simulink model "fft_wideband_real"  (R2012b)
settings: Solver=ode45  StartTime=0.0  StopTime=19999  RelTol=1e-3
undefined symbols (not defined in the file): fft_wideband_real_shift_schedule_user_data_out
libraries: xbsIndex_r4 x8703, xbsReplacements_r4 x36, xps_library x24, dspsigops x16, simulink_xsg_bridge x1
(part 7 of 51)

== system fft_wideband_real/fft_wideband_real/phase_mult/cmult_1 ==
  a : Inport
  b : Inport  Port=2
  AddSub : xbsIndex_r4/AddSub  mode=Subtraction  use_carryin=off  use_carryout=off  en=off  latency=2  precision=Full  arith_type=Unsigned  n_bits=16  bin_pt=14  quantization=Truncate  overflow=Wrap  dbl_ovrd=off  use_behavioral_HDL=on  hw_selection=Fabric  pipelined=off  block_type=addsub
  AddSub1 : xbsIndex_r4/AddSub  mode=Addition  use_carryin=off  use_carryout=off  en=off  latency=2  precision=Full  arith_type=Unsigned  n_bits=16  bin_pt=14  quantization=Truncate  overflow=Wrap  dbl_ovrd=off  use_behavioral_HDL=on  hw_selection=Fabric  pipelined=off  block_type=addsub
  a_input_c_to_ri : Subsystem
      settings: AttributesFormatString=18_17 r/i
  b_input_c_to_ri : Subsystem
      settings: AttributesFormatString=18_17 r/i
  c_output_ri_to_c : Subsystem
  convert0 : xbsIndex_r4/Convert  gui_display_data_type=Fixed-point  arith_type="Signed  (2's comp)"  n_bits=18  bin_pt=17  float_type=Single  exp_bits=8  fraction_bits=24  quantization="Round  (unbiased: +/- Inf)"  overflow=Saturate  en=off  latency=1  dbl_ovrd=off  pipeline=on  block_type=convert
  convert1 : xbsIndex_r4/Convert  gui_display_data_type=Fixed-point  arith_type="Signed  (2's comp)"  n_bits=18  bin_pt=17  float_type=Single  exp_bits=8  fraction_bits=24  quantization="Round  (unbiased: +/- Inf)"  overflow=Saturate  en=off  latency=1  dbl_ovrd=off  pipeline=on  block_type=convert
  mults : Subsystem
  c : Outport
  wires:
  a_input_c_to_ri/1(re) -> mults/7(a4), mults/1(a1)  "a_re"
  b_input_c_to_ri/1(re) -> mults/6(b3), mults/2(b1)  "b_re"
  a_input_c_to_ri/2(im) -> mults/5(a3), mults/3(a2)  "a_im"
  b_input_c_to_ri/2(im) -> mults/8(b4), mults/4(b2)  "b_im"
  convert1/1 -> c_output_ri_to_c/2(im)  "c_im"
  AddSub1/1 -> convert1/1
  convert0/1 -> c_output_ri_to_c/1(re)  "c_re"
  AddSub/1 -> convert0/1
  mults/4(c4) -> AddSub1/2
  mults/3(c3) -> AddSub1/1
  mults/2(c2) -> AddSub/2
  mults/1(c1) -> AddSub/1
  c_output_ri_to_c/1(c) -> c/1
  b/1 -> b_input_c_to_ri/1(c)
  a/1 -> a_input_c_to_ri/1(c)

== system fft_wideband_real/fft_wideband_real/phase_mult/cmult_10 ==
  a : Inport
  b : Inport  Port=2
  AddSub : xbsIndex_r4/AddSub  mode=Subtraction  use_carryin=off  use_carryout=off  en=off  latency=2  precision=Full  arith_type=Unsigned  n_bits=16  bin_pt=14  quantization=Truncate  overflow=Wrap  dbl_ovrd=off  use_behavioral_HDL=on  hw_selection=Fabric  pipelined=off  block_type=addsub
  AddSub1 : xbsIndex_r4/AddSub  mode=Addition  use_carryin=off  use_carryout=off  en=off  latency=2  precision=Full  arith_type=Unsigned  n_bits=16  bin_pt=14  quantization=Truncate  overflow=Wrap  dbl_ovrd=off  use_behavioral_HDL=on  hw_selection=Fabric  pipelined=off  block_type=addsub
  a_input_c_to_ri : Subsystem
      settings: AttributesFormatString=18_17 r/i
  b_input_c_to_ri : Subsystem
      settings: AttributesFormatString=18_17 r/i
  c_output_ri_to_c : Subsystem
  convert0 : xbsIndex_r4/Convert  gui_display_data_type=Fixed-point  arith_type="Signed  (2's comp)"  n_bits=18  bin_pt=17  float_type=Single  exp_bits=8  fraction_bits=24  quantization="Round  (unbiased: +/- Inf)"  overflow=Saturate  en=off  latency=1  dbl_ovrd=off  pipeline=on  block_type=convert
  convert1 : xbsIndex_r4/Convert  gui_display_data_type=Fixed-point  arith_type="Signed  (2's comp)"  n_bits=18  bin_pt=17  float_type=Single  exp_bits=8  fraction_bits=24  quantization="Round  (unbiased: +/- Inf)"  overflow=Saturate  en=off  latency=1  dbl_ovrd=off  pipeline=on  block_type=convert
  mults : Subsystem
  c : Outport
  wires:
  a_input_c_to_ri/1(re) -> mults/7(a4), mults/1(a1)  "a_re"
  b_input_c_to_ri/1(re) -> mults/6(b3), mults/2(b1)  "b_re"
  a_input_c_to_ri/2(im) -> mults/5(a3), mults/3(a2)  "a_im"
  b_input_c_to_ri/2(im) -> mults/8(b4), mults/4(b2)  "b_im"
  convert1/1 -> c_output_ri_to_c/2(im)  "c_im"
  AddSub1/1 -> convert1/1
  convert0/1 -> c_output_ri_to_c/1(re)  "c_re"
  AddSub/1 -> convert0/1
  mults/4(c4) -> AddSub1/2
  mults/3(c3) -> AddSub1/1
  mults/2(c2) -> AddSub/2
  mults/1(c1) -> AddSub/1
  c_output_ri_to_c/1(c) -> c/1
  b/1 -> b_input_c_to_ri/1(c)
  a/1 -> a_input_c_to_ri/1(c)

== system fft_wideband_real/fft_wideband_real/phase_mult/cmult_11 ==
  a : Inport
  b : Inport  Port=2
  AddSub : xbsIndex_r4/AddSub  mode=Subtraction  use_carryin=off  use_carryout=off  en=off  latency=2  precision=Full  arith_type=Unsigned  n_bits=16  bin_pt=14  quantization=Truncate  overflow=Wrap  dbl_ovrd=off  use_behavioral_HDL=on  hw_selection=Fabric  pipelined=off  block_type=addsub
  AddSub1 : xbsIndex_r4/AddSub  mode=Addition  use_carryin=off  use_carryout=off  en=off  latency=2  precision=Full  arith_type=Unsigned  n_bits=16  bin_pt=14  quantization=Truncate  overflow=Wrap  dbl_ovrd=off  use_behavioral_HDL=on  hw_selection=Fabric  pipelined=off  block_type=addsub
  a_input_c_to_ri : Subsystem
      settings: AttributesFormatString=18_17 r/i
  b_input_c_to_ri : Subsystem
      settings: AttributesFormatString=18_17 r/i
  c_output_ri_to_c : Subsystem
  convert0 : xbsIndex_r4/Convert  gui_display_data_type=Fixed-point  arith_type="Signed  (2's comp)"  n_bits=18  bin_pt=17  float_type=Single  exp_bits=8  fraction_bits=24  quantization="Round  (unbiased: +/- Inf)"  overflow=Saturate  en=off  latency=1  dbl_ovrd=off  pipeline=on  block_type=convert
  convert1 : xbsIndex_r4/Convert  gui_display_data_type=Fixed-point  arith_type="Signed  (2's comp)"  n_bits=18  bin_pt=17  float_type=Single  exp_bits=8  fraction_bits=24  quantization="Round  (unbiased: +/- Inf)"  overflow=Saturate  en=off  latency=1  dbl_ovrd=off  pipeline=on  block_type=convert
  mults : Subsystem
  c : Outport
  wires:
  a_input_c_to_ri/1(re) -> mults/7(a4), mults/1(a1)  "a_re"
  b_input_c_to_ri/1(re) -> mults/6(b3), mults/2(b1)  "b_re"
  a_input_c_to_ri/2(im) -> mults/5(a3), mults/3(a2)  "a_im"
  b_input_c_to_ri/2(im) -> mults/8(b4), mults/4(b2)  "b_im"
  convert1/1 -> c_output_ri_to_c/2(im)  "c_im"
  AddSub1/1 -> convert1/1
  convert0/1 -> c_output_ri_to_c/1(re)  "c_re"
  AddSub/1 -> convert0/1
  mults/4(c4) -> AddSub1/2
  mults/3(c3) -> AddSub1/1
  mults/2(c2) -> AddSub/2
  mults/1(c1) -> AddSub/1
  c_output_ri_to_c/1(c) -> c/1
  b/1 -> b_input_c_to_ri/1(c)
  a/1 -> a_input_c_to_ri/1(c)

== system fft_wideband_real/fft_wideband_real/phase_mult/cmult_12 ==
  a : Inport
  b : Inport  Port=2
  AddSub : xbsIndex_r4/AddSub  mode=Subtraction  use_carryin=off  use_carryout=off  en=off  latency=2  precision=Full  arith_type=Unsigned  n_bits=16  bin_pt=14  quantization=Truncate  overflow=Wrap  dbl_ovrd=off  use_behavioral_HDL=on  hw_selection=Fabric  pipelined=off  block_type=addsub
  AddSub1 : xbsIndex_r4/AddSub  mode=Addition  use_carryin=off  use_carryout=off  en=off  latency=2  precision=Full  arith_type=Unsigned  n_bits=16  bin_pt=14  quantization=Truncate  overflow=Wrap  dbl_ovrd=off  use_behavioral_HDL=on  hw_selection=Fabric  pipelined=off  block_type=addsub
  a_input_c_to_ri : Subsystem
      settings: AttributesFormatString=18_17 r/i
  b_input_c_to_ri : Subsystem
      settings: AttributesFormatString=18_17 r/i
  c_output_ri_to_c : Subsystem
  convert0 : xbsIndex_r4/Convert  gui_display_data_type=Fixed-point  arith_type="Signed  (2's comp)"  n_bits=18  bin_pt=17  float_type=Single  exp_bits=8  fraction_bits=24  quantization="Round  (unbiased: +/- Inf)"  overflow=Saturate  en=off  latency=1  dbl_ovrd=off  pipeline=on  block_type=convert
  convert1 : xbsIndex_r4/Convert  gui_display_data_type=Fixed-point  arith_type="Signed  (2's comp)"  n_bits=18  bin_pt=17  float_type=Single  exp_bits=8  fraction_bits=24  quantization="Round  (unbiased: +/- Inf)"  overflow=Saturate  en=off  latency=1  dbl_ovrd=off  pipeline=on  block_type=convert
  mults : Subsystem
  c : Outport
  wires:
  a_input_c_to_ri/1(re) -> mults/7(a4), mults/1(a1)  "a_re"
  b_input_c_to_ri/1(re) -> mults/6(b3), mults/2(b1)  "b_re"
  a_input_c_to_ri/2(im) -> mults/5(a3), mults/3(a2)  "a_im"
  b_input_c_to_ri/2(im) -> mults/8(b4), mults/4(b2)  "b_im"
  convert1/1 -> c_output_ri_to_c/2(im)  "c_im"
  AddSub1/1 -> convert1/1
  convert0/1 -> c_output_ri_to_c/1(re)  "c_re"
  AddSub/1 -> convert0/1
  mults/4(c4) -> AddSub1/2
  mults/3(c3) -> AddSub1/1
  mults/2(c2) -> AddSub/2
  mults/1(c1) -> AddSub/1
  c_output_ri_to_c/1(c) -> c/1
  b/1 -> b_input_c_to_ri/1(c)
  a/1 -> a_input_c_to_ri/1(c)

== system fft_wideband_real/fft_wideband_real/phase_mult/cmult_13 ==
  a : Inport
  b : Inport  Port=2
  AddSub : xbsIndex_r4/AddSub  mode=Subtraction  use_carryin=off  use_carryout=off  en=off  latency=2  precision=Full  arith_type=Unsigned  n_bits=16  bin_pt=14  quantization=Truncate  overflow=Wrap  dbl_ovrd=off  use_behavioral_HDL=on  hw_selection=Fabric  pipelined=off  block_type=addsub
  AddSub1 : xbsIndex_r4/AddSub  mode=Addition  use_carryin=off  use_carryout=off  en=off  latency=2  precision=Full  arith_type=Unsigned  n_bits=16  bin_pt=14  quantization=Truncate  overflow=Wrap  dbl_ovrd=off  use_behavioral_HDL=on  hw_selection=Fabric  pipelined=off  block_type=addsub
  a_input_c_to_ri : Subsystem
      settings: AttributesFormatString=18_17 r/i
  b_input_c_to_ri : Subsystem
      settings: AttributesFormatString=18_17 r/i
  c_output_ri_to_c : Subsystem
  convert0 : xbsIndex_r4/Convert  gui_display_data_type=Fixed-point  arith_type="Signed  (2's comp)"  n_bits=18  bin_pt=17  float_type=Single  exp_bits=8  fraction_bits=24  quantization="Round  (unbiased: +/- Inf)"  overflow=Saturate  en=off  latency=1  dbl_ovrd=off  pipeline=on  block_type=convert
  convert1 : xbsIndex_r4/Convert  gui_display_data_type=Fixed-point  arith_type="Signed  (2's comp)"  n_bits=18  bin_pt=17  float_type=Single  exp_bits=8  fraction_bits=24  quantization="Round  (unbiased: +/- Inf)"  overflow=Saturate  en=off  latency=1  dbl_ovrd=off  pipeline=on  block_type=convert
  mults : Subsystem
  c : Outport
  wires:
  a_input_c_to_ri/1(re) -> mults/7(a4), mults/1(a1)  "a_re"
  b_input_c_to_ri/1(re) -> mults/6(b3), mults/2(b1)  "b_re"
  a_input_c_to_ri/2(im) -> mults/5(a3), mults/3(a2)  "a_im"
  b_input_c_to_ri/2(im) -> mults/8(b4), mults/4(b2)  "b_im"
  convert1/1 -> c_output_ri_to_c/2(im)  "c_im"
  AddSub1/1 -> convert1/1
  convert0/1 -> c_output_ri_to_c/1(re)  "c_re"
  AddSub/1 -> convert0/1
  mults/4(c4) -> AddSub1/2
  mults/3(c3) -> AddSub1/1
  mults/2(c2) -> AddSub/2
  mults/1(c1) -> AddSub/1
  c_output_ri_to_c/1(c) -> c/1
  b/1 -> b_input_c_to_ri/1(c)
  a/1 -> a_input_c_to_ri/1(c)

== system fft_wideband_real/fft_wideband_real/phase_mult/cmult_14 ==
  a : Inport
  b : Inport  Port=2
  AddSub : xbsIndex_r4/AddSub  mode=Subtraction  use_carryin=off  use_carryout=off  en=off  latency=2  precision=Full  arith_type=Unsigned  n_bits=16  bin_pt=14  quantization=Truncate  overflow=Wrap  dbl_ovrd=off  use_behavioral_HDL=on  hw_selection=Fabric  pipelined=off  block_type=addsub
  AddSub1 : xbsIndex_r4/AddSub  mode=Addition  use_carryin=off  use_carryout=off  en=off  latency=2  precision=Full  arith_type=Unsigned  n_bits=16  bin_pt=14  quantization=Truncate  overflow=Wrap  dbl_ovrd=off  use_behavioral_HDL=on  hw_selection=Fabric  pipelined=off  block_type=addsub
  a_input_c_to_ri : Subsystem
      settings: AttributesFormatString=18_17 r/i
  b_input_c_to_ri : Subsystem
      settings: AttributesFormatString=18_17 r/i
  c_output_ri_to_c : Subsystem
  convert0 : xbsIndex_r4/Convert  gui_display_data_type=Fixed-point  arith_type="Signed  (2's comp)"  n_bits=18  bin_pt=17  float_type=Single  exp_bits=8  fraction_bits=24  quantization="Round  (unbiased: +/- Inf)"  overflow=Saturate  en=off  latency=1  dbl_ovrd=off  pipeline=on  block_type=convert
  convert1 : xbsIndex_r4/Convert  gui_display_data_type=Fixed-point  arith_type="Signed  (2's comp)"  n_bits=18  bin_pt=17  float_type=Single  exp_bits=8  fraction_bits=24  quantization="Round  (unbiased: +/- Inf)"  overflow=Saturate  en=off  latency=1  dbl_ovrd=off  pipeline=on  block_type=convert
  mults : Subsystem
  c : Outport
  wires:
  a_input_c_to_ri/1(re) -> mults/7(a4), mults/1(a1)  "a_re"
  b_input_c_to_ri/1(re) -> mults/6(b3), mults/2(b1)  "b_re"
  a_input_c_to_ri/2(im) -> mults/5(a3), mults/3(a2)  "a_im"
  b_input_c_to_ri/2(im) -> mults/8(b4), mults/4(b2)  "b_im"
  convert1/1 -> c_output_ri_to_c/2(im)  "c_im"
  AddSub1/1 -> convert1/1
  convert0/1 -> c_output_ri_to_c/1(re)  "c_re"
  AddSub/1 -> convert0/1
  mults/4(c4) -> AddSub1/2
  mults/3(c3) -> AddSub1/1
  mults/2(c2) -> AddSub/2
  mults/1(c1) -> AddSub/1
  c_output_ri_to_c/1(c) -> c/1
  b/1 -> b_input_c_to_ri/1(c)
  a/1 -> a_input_c_to_ri/1(c)

== system fft_wideband_real/fft_wideband_real/phase_mult/cmult_15 ==
  a : Inport
  b : Inport  Port=2
  AddSub : xbsIndex_r4/AddSub  mode=Subtraction  use_carryin=off  use_carryout=off  en=off  latency=2  precision=Full  arith_type=Unsigned  n_bits=16  bin_pt=14  quantization=Truncate  overflow=Wrap  dbl_ovrd=off  use_behavioral_HDL=on  hw_selection=Fabric  pipelined=off  block_type=addsub
  AddSub1 : xbsIndex_r4/AddSub  mode=Addition  use_carryin=off  use_carryout=off  en=off  latency=2  precision=Full  arith_type=Unsigned  n_bits=16  bin_pt=14  quantization=Truncate  overflow=Wrap  dbl_ovrd=off  use_behavioral_HDL=on  hw_selection=Fabric  pipelined=off  block_type=addsub
  a_input_c_to_ri : Subsystem
      settings: AttributesFormatString=18_17 r/i
  b_input_c_to_ri : Subsystem
      settings: AttributesFormatString=18_17 r/i
  c_output_ri_to_c : Subsystem
  convert0 : xbsIndex_r4/Convert  gui_display_data_type=Fixed-point  arith_type="Signed  (2's comp)"  n_bits=18  bin_pt=17  float_type=Single  exp_bits=8  fraction_bits=24  quantization="Round  (unbiased: +/- Inf)"  overflow=Saturate  en=off  latency=1  dbl_ovrd=off  pipeline=on  block_type=convert
  convert1 : xbsIndex_r4/Convert  gui_display_data_type=Fixed-point  arith_type="Signed  (2's comp)"  n_bits=18  bin_pt=17  float_type=Single  exp_bits=8  fraction_bits=24  quantization="Round  (unbiased: +/- Inf)"  overflow=Saturate  en=off  latency=1  dbl_ovrd=off  pipeline=on  block_type=convert
  mults : Subsystem
  c : Outport
  wires:
  a_input_c_to_ri/1(re) -> mults/7(a4), mults/1(a1)  "a_re"
  b_input_c_to_ri/1(re) -> mults/6(b3), mults/2(b1)  "b_re"
  a_input_c_to_ri/2(im) -> mults/5(a3), mults/3(a2)  "a_im"
  b_input_c_to_ri/2(im) -> mults/8(b4), mults/4(b2)  "b_im"
  convert1/1 -> c_output_ri_to_c/2(im)  "c_im"
  AddSub1/1 -> convert1/1
  convert0/1 -> c_output_ri_to_c/1(re)  "c_re"
  AddSub/1 -> convert0/1
  mults/4(c4) -> AddSub1/2
  mults/3(c3) -> AddSub1/1
  mults/2(c2) -> AddSub/2
  mults/1(c1) -> AddSub/1
  c_output_ri_to_c/1(c) -> c/1
  b/1 -> b_input_c_to_ri/1(c)
  a/1 -> a_input_c_to_ri/1(c)

== system fft_wideband_real/fft_wideband_real/phase_mult/cmult_16 ==
  a : Inport
  b : Inport  Port=2
  AddSub : xbsIndex_r4/AddSub  mode=Subtraction  use_carryin=off  use_carryout=off  en=off  latency=2  precision=Full  arith_type=Unsigned  n_bits=16  bin_pt=14  quantization=Truncate  overflow=Wrap  dbl_ovrd=off  use_behavioral_HDL=on  hw_selection=Fabric  pipelined=off  block_type=addsub
  AddSub1 : xbsIndex_r4/AddSub  mode=Addition  use_carryin=off  use_carryout=off  en=off  latency=2  precision=Full  arith_type=Unsigned  n_bits=16  bin_pt=14  quantization=Truncate  overflow=Wrap  dbl_ovrd=off  use_behavioral_HDL=on  hw_selection=Fabric  pipelined=off  block_type=addsub
  a_input_c_to_ri : Subsystem
      settings: AttributesFormatString=18_17 r/i
  b_input_c_to_ri : Subsystem
      settings: AttributesFormatString=18_17 r/i
  c_output_ri_to_c : Subsystem
  convert0 : xbsIndex_r4/Convert  gui_display_data_type=Fixed-point  arith_type="Signed  (2's comp)"  n_bits=18  bin_pt=17  float_type=Single  exp_bits=8  fraction_bits=24  quantization="Round  (unbiased: +/- Inf)"  overflow=Saturate  en=off  latency=1  dbl_ovrd=off  pipeline=on  block_type=convert
  convert1 : xbsIndex_r4/Convert  gui_display_data_type=Fixed-point  arith_type="Signed  (2's comp)"  n_bits=18  bin_pt=17  float_type=Single  exp_bits=8  fraction_bits=24  quantization="Round  (unbiased: +/- Inf)"  overflow=Saturate  en=off  latency=1  dbl_ovrd=off  pipeline=on  block_type=convert
  mults : Subsystem
  c : Outport
  wires:
  a_input_c_to_ri/1(re) -> mults/7(a4), mults/1(a1)  "a_re"
  b_input_c_to_ri/1(re) -> mults/6(b3), mults/2(b1)  "b_re"
  a_input_c_to_ri/2(im) -> mults/5(a3), mults/3(a2)  "a_im"
  b_input_c_to_ri/2(im) -> mults/8(b4), mults/4(b2)  "b_im"
  convert1/1 -> c_output_ri_to_c/2(im)  "c_im"
  AddSub1/1 -> convert1/1
  convert0/1 -> c_output_ri_to_c/1(re)  "c_re"
  AddSub/1 -> convert0/1
  mults/4(c4) -> AddSub1/2
  mults/3(c3) -> AddSub1/1
  mults/2(c2) -> AddSub/2
  mults/1(c1) -> AddSub/1
  c_output_ri_to_c/1(c) -> c/1
  b/1 -> b_input_c_to_ri/1(c)
  a/1 -> a_input_c_to_ri/1(c)

== system fft_wideband_real/fft_wideband_real/phase_mult/cmult_2 ==
  a : Inport
  b : Inport  Port=2
  AddSub : xbsIndex_r4/AddSub  mode=Subtraction  use_carryin=off  use_carryout=off  en=off  latency=2  precision=Full  arith_type=Unsigned  n_bits=16  bin_pt=14  quantization=Truncate  overflow=Wrap  dbl_ovrd=off  use_behavioral_HDL=on  hw_selection=Fabric  pipelined=off  block_type=addsub
  AddSub1 : xbsIndex_r4/AddSub  mode=Addition  use_carryin=off  use_carryout=off  en=off  latency=2  precision=Full  arith_type=Unsigned  n_bits=16  bin_pt=14  quantization=Truncate  overflow=Wrap  dbl_ovrd=off  use_behavioral_HDL=on  hw_selection=Fabric  pipelined=off  block_type=addsub
  a_input_c_to_ri : Subsystem
      settings: AttributesFormatString=18_17 r/i
  b_input_c_to_ri : Subsystem
      settings: AttributesFormatString=18_17 r/i
  c_output_ri_to_c : Subsystem
  convert0 : xbsIndex_r4/Convert  gui_display_data_type=Fixed-point  arith_type="Signed  (2's comp)"  n_bits=18  bin_pt=17  float_type=Single  exp_bits=8  fraction_bits=24  quantization="Round  (unbiased: +/- Inf)"  overflow=Saturate  en=off  latency=1  dbl_ovrd=off  pipeline=on  block_type=convert
  convert1 : xbsIndex_r4/Convert  gui_display_data_type=Fixed-point  arith_type="Signed  (2's comp)"  n_bits=18  bin_pt=17  float_type=Single  exp_bits=8  fraction_bits=24  quantization="Round  (unbiased: +/- Inf)"  overflow=Saturate  en=off  latency=1  dbl_ovrd=off  pipeline=on  block_type=convert
  mults : Subsystem
  c : Outport
  wires:
  a_input_c_to_ri/1(re) -> mults/7(a4), mults/1(a1)  "a_re"
  b_input_c_to_ri/1(re) -> mults/6(b3), mults/2(b1)  "b_re"
  a_input_c_to_ri/2(im) -> mults/5(a3), mults/3(a2)  "a_im"
  b_input_c_to_ri/2(im) -> mults/8(b4), mults/4(b2)  "b_im"
  convert1/1 -> c_output_ri_to_c/2(im)  "c_im"
  AddSub1/1 -> convert1/1
  convert0/1 -> c_output_ri_to_c/1(re)  "c_re"
  AddSub/1 -> convert0/1
  mults/4(c4) -> AddSub1/2
  mults/3(c3) -> AddSub1/1
  mults/2(c2) -> AddSub/2
  mults/1(c1) -> AddSub/1
  c_output_ri_to_c/1(c) -> c/1
  b/1 -> b_input_c_to_ri/1(c)
  a/1 -> a_input_c_to_ri/1(c)

== system fft_wideband_real/fft_wideband_real/phase_mult/cmult_3 ==
  a : Inport
  b : Inport  Port=2
  AddSub : xbsIndex_r4/AddSub  mode=Subtraction  use_carryin=off  use_carryout=off  en=off  latency=2  precision=Full  arith_type=Unsigned  n_bits=16  bin_pt=14  quantization=Truncate  overflow=Wrap  dbl_ovrd=off  use_behavioral_HDL=on  hw_selection=Fabric  pipelined=off  block_type=addsub
  AddSub1 : xbsIndex_r4/AddSub  mode=Addition  use_carryin=off  use_carryout=off  en=off  latency=2  precision=Full  arith_type=Unsigned  n_bits=16  bin_pt=14  quantization=Truncate  overflow=Wrap  dbl_ovrd=off  use_behavioral_HDL=on  hw_selection=Fabric  pipelined=off  block_type=addsub
  a_input_c_to_ri : Subsystem
      settings: AttributesFormatString=18_17 r/i
  b_input_c_to_ri : Subsystem
      settings: AttributesFormatString=18_17 r/i
  c_output_ri_to_c : Subsystem
  convert0 : xbsIndex_r4/Convert  gui_display_data_type=Fixed-point  arith_type="Signed  (2's comp)"  n_bits=18  bin_pt=17  float_type=Single  exp_bits=8  fraction_bits=24  quantization="Round  (unbiased: +/- Inf)"  overflow=Saturate  en=off  latency=1  dbl_ovrd=off  pipeline=on  block_type=convert
  convert1 : xbsIndex_r4/Convert  gui_display_data_type=Fixed-point  arith_type="Signed  (2's comp)"  n_bits=18  bin_pt=17  float_type=Single  exp_bits=8  fraction_bits=24  quantization="Round  (unbiased: +/- Inf)"  overflow=Saturate  en=off  latency=1  dbl_ovrd=off  pipeline=on  block_type=convert
  mults : Subsystem
  c : Outport
  wires:
  a_input_c_to_ri/1(re) -> mults/7(a4), mults/1(a1)  "a_re"
  b_input_c_to_ri/1(re) -> mults/6(b3), mults/2(b1)  "b_re"
  a_input_c_to_ri/2(im) -> mults/5(a3), mults/3(a2)  "a_im"
  b_input_c_to_ri/2(im) -> mults/8(b4), mults/4(b2)  "b_im"
  convert1/1 -> c_output_ri_to_c/2(im)  "c_im"
  AddSub1/1 -> convert1/1
  convert0/1 -> c_output_ri_to_c/1(re)  "c_re"
  AddSub/1 -> convert0/1
  mults/4(c4) -> AddSub1/2
  mults/3(c3) -> AddSub1/1
  mults/2(c2) -> AddSub/2
  mults/1(c1) -> AddSub/1
  c_output_ri_to_c/1(c) -> c/1
  b/1 -> b_input_c_to_ri/1(c)
  a/1 -> a_input_c_to_ri/1(c)

== system fft_wideband_real/fft_wideband_real/phase_mult/cmult_4 ==
  a : Inport
  b : Inport  Port=2
  AddSub : xbsIndex_r4/AddSub  mode=Subtraction  use_carryin=off  use_carryout=off  en=off  latency=2  precision=Full  arith_type=Unsigned  n_bits=16  bin_pt=14  quantization=Truncate  overflow=Wrap  dbl_ovrd=off  use_behavioral_HDL=on  hw_selection=Fabric  pipelined=off  block_type=addsub
  AddSub1 : xbsIndex_r4/AddSub  mode=Addition  use_carryin=off  use_carryout=off  en=off  latency=2  precision=Full  arith_type=Unsigned  n_bits=16  bin_pt=14  quantization=Truncate  overflow=Wrap  dbl_ovrd=off  use_behavioral_HDL=on  hw_selection=Fabric  pipelined=off  block_type=addsub
  a_input_c_to_ri : Subsystem
      settings: AttributesFormatString=18_17 r/i
  b_input_c_to_ri : Subsystem
      settings: AttributesFormatString=18_17 r/i
  c_output_ri_to_c : Subsystem
  convert0 : xbsIndex_r4/Convert  gui_display_data_type=Fixed-point  arith_type="Signed  (2's comp)"  n_bits=18  bin_pt=17  float_type=Single  exp_bits=8  fraction_bits=24  quantization="Round  (unbiased: +/- Inf)"  overflow=Saturate  en=off  latency=1  dbl_ovrd=off  pipeline=on  block_type=convert
  convert1 : xbsIndex_r4/Convert  gui_display_data_type=Fixed-point  arith_type="Signed  (2's comp)"  n_bits=18  bin_pt=17  float_type=Single  exp_bits=8  fraction_bits=24  quantization="Round  (unbiased: +/- Inf)"  overflow=Saturate  en=off  latency=1  dbl_ovrd=off  pipeline=on  block_type=convert
  mults : Subsystem
  c : Outport
  wires:
  a_input_c_to_ri/1(re) -> mults/7(a4), mults/1(a1)  "a_re"
  b_input_c_to_ri/1(re) -> mults/6(b3), mults/2(b1)  "b_re"
  a_input_c_to_ri/2(im) -> mults/5(a3), mults/3(a2)  "a_im"
  b_input_c_to_ri/2(im) -> mults/8(b4), mults/4(b2)  "b_im"
  convert1/1 -> c_output_ri_to_c/2(im)  "c_im"
  AddSub1/1 -> convert1/1
  convert0/1 -> c_output_ri_to_c/1(re)  "c_re"
  AddSub/1 -> convert0/1
  mults/4(c4) -> AddSub1/2
  mults/3(c3) -> AddSub1/1
  mults/2(c2) -> AddSub/2
  mults/1(c1) -> AddSub/1
  c_output_ri_to_c/1(c) -> c/1
  b/1 -> b_input_c_to_ri/1(c)
  a/1 -> a_input_c_to_ri/1(c)

== system fft_wideband_real/fft_wideband_real/phase_mult/cmult_5 ==
  a : Inport
  b : Inport  Port=2
  AddSub : xbsIndex_r4/AddSub  mode=Subtraction  use_carryin=off  use_carryout=off  en=off  latency=2  precision=Full  arith_type=Unsigned  n_bits=16  bin_pt=14  quantization=Truncate  overflow=Wrap  dbl_ovrd=off  use_behavioral_HDL=on  hw_selection=Fabric  pipelined=off  block_type=addsub
  AddSub1 : xbsIndex_r4/AddSub  mode=Addition  use_carryin=off  use_carryout=off  en=off  latency=2  precision=Full  arith_type=Unsigned  n_bits=16  bin_pt=14  quantization=Truncate  overflow=Wrap  dbl_ovrd=off  use_behavioral_HDL=on  hw_selection=Fabric  pipelined=off  block_type=addsub
  a_input_c_to_ri : Subsystem
      settings: AttributesFormatString=18_17 r/i
  b_input_c_to_ri : Subsystem
      settings: AttributesFormatString=18_17 r/i
  c_output_ri_to_c : Subsystem
  convert0 : xbsIndex_r4/Convert  gui_display_data_type=Fixed-point  arith_type="Signed  (2's comp)"  n_bits=18  bin_pt=17  float_type=Single  exp_bits=8  fraction_bits=24  quantization="Round  (unbiased: +/- Inf)"  overflow=Saturate  en=off  latency=1  dbl_ovrd=off  pipeline=on  block_type=convert
  convert1 : xbsIndex_r4/Convert  gui_display_data_type=Fixed-point  arith_type="Signed  (2's comp)"  n_bits=18  bin_pt=17  float_type=Single  exp_bits=8  fraction_bits=24  quantization="Round  (unbiased: +/- Inf)"  overflow=Saturate  en=off  latency=1  dbl_ovrd=off  pipeline=on  block_type=convert
  mults : Subsystem
  c : Outport
  wires:
  a_input_c_to_ri/1(re) -> mults/7(a4), mults/1(a1)  "a_re"
  b_input_c_to_ri/1(re) -> mults/6(b3), mults/2(b1)  "b_re"
  a_input_c_to_ri/2(im) -> mults/5(a3), mults/3(a2)  "a_im"
  b_input_c_to_ri/2(im) -> mults/8(b4), mults/4(b2)  "b_im"
  convert1/1 -> c_output_ri_to_c/2(im)  "c_im"
  AddSub1/1 -> convert1/1
  convert0/1 -> c_output_ri_to_c/1(re)  "c_re"
  AddSub/1 -> convert0/1
  mults/4(c4) -> AddSub1/2
  mults/3(c3) -> AddSub1/1
  mults/2(c2) -> AddSub/2
  mults/1(c1) -> AddSub/1
  c_output_ri_to_c/1(c) -> c/1
  b/1 -> b_input_c_to_ri/1(c)
  a/1 -> a_input_c_to_ri/1(c)

== system fft_wideband_real/fft_wideband_real/phase_mult/cmult_6 ==
  a : Inport
  b : Inport  Port=2
  AddSub : xbsIndex_r4/AddSub  mode=Subtraction  use_carryin=off  use_carryout=off  en=off  latency=2  precision=Full  arith_type=Unsigned  n_bits=16  bin_pt=14  quantization=Truncate  overflow=Wrap  dbl_ovrd=off  use_behavioral_HDL=on  hw_selection=Fabric  pipelined=off  block_type=addsub
  AddSub1 : xbsIndex_r4/AddSub  mode=Addition  use_carryin=off  use_carryout=off  en=off  latency=2  precision=Full  arith_type=Unsigned  n_bits=16  bin_pt=14  quantization=Truncate  overflow=Wrap  dbl_ovrd=off  use_behavioral_HDL=on  hw_selection=Fabric  pipelined=off  block_type=addsub
  a_input_c_to_ri : Subsystem
      settings: AttributesFormatString=18_17 r/i
  b_input_c_to_ri : Subsystem
      settings: AttributesFormatString=18_17 r/i
  c_output_ri_to_c : Subsystem
  convert0 : xbsIndex_r4/Convert  gui_display_data_type=Fixed-point  arith_type="Signed  (2's comp)"  n_bits=18  bin_pt=17  float_type=Single  exp_bits=8  fraction_bits=24  quantization="Round  (unbiased: +/- Inf)"  overflow=Saturate  en=off  latency=1  dbl_ovrd=off  pipeline=on  block_type=convert
  convert1 : xbsIndex_r4/Convert  gui_display_data_type=Fixed-point  arith_type="Signed  (2's comp)"  n_bits=18  bin_pt=17  float_type=Single  exp_bits=8  fraction_bits=24  quantization="Round  (unbiased: +/- Inf)"  overflow=Saturate  en=off  latency=1  dbl_ovrd=off  pipeline=on  block_type=convert
  mults : Subsystem
  c : Outport
  wires:
  a_input_c_to_ri/1(re) -> mults/7(a4), mults/1(a1)  "a_re"
  b_input_c_to_ri/1(re) -> mults/6(b3), mults/2(b1)  "b_re"
  a_input_c_to_ri/2(im) -> mults/5(a3), mults/3(a2)  "a_im"
  b_input_c_to_ri/2(im) -> mults/8(b4), mults/4(b2)  "b_im"
  convert1/1 -> c_output_ri_to_c/2(im)  "c_im"
  AddSub1/1 -> convert1/1
  convert0/1 -> c_output_ri_to_c/1(re)  "c_re"
  AddSub/1 -> convert0/1
  mults/4(c4) -> AddSub1/2
  mults/3(c3) -> AddSub1/1
  mults/2(c2) -> AddSub/2
  mults/1(c1) -> AddSub/1
  c_output_ri_to_c/1(c) -> c/1
  b/1 -> b_input_c_to_ri/1(c)
  a/1 -> a_input_c_to_ri/1(c)

== system fft_wideband_real/fft_wideband_real/phase_mult/cmult_7 ==
  a : Inport
  b : Inport  Port=2
  AddSub : xbsIndex_r4/AddSub  mode=Subtraction  use_carryin=off  use_carryout=off  en=off  latency=2  precision=Full  arith_type=Unsigned  n_bits=16  bin_pt=14  quantization=Truncate  overflow=Wrap  dbl_ovrd=off  use_behavioral_HDL=on  hw_selection=Fabric  pipelined=off  block_type=addsub
  AddSub1 : xbsIndex_r4/AddSub  mode=Addition  use_carryin=off  use_carryout=off  en=off  latency=2  precision=Full  arith_type=Unsigned  n_bits=16  bin_pt=14  quantization=Truncate  overflow=Wrap  dbl_ovrd=off  use_behavioral_HDL=on  hw_selection=Fabric  pipelined=off  block_type=addsub
  a_input_c_to_ri : Subsystem
      settings: AttributesFormatString=18_17 r/i
  b_input_c_to_ri : Subsystem
      settings: AttributesFormatString=18_17 r/i
  c_output_ri_to_c : Subsystem
  convert0 : xbsIndex_r4/Convert  gui_display_data_type=Fixed-point  arith_type="Signed  (2's comp)"  n_bits=18  bin_pt=17  float_type=Single  exp_bits=8  fraction_bits=24  quantization="Round  (unbiased: +/- Inf)"  overflow=Saturate  en=off  latency=1  dbl_ovrd=off  pipeline=on  block_type=convert
  convert1 : xbsIndex_r4/Convert  gui_display_data_type=Fixed-point  arith_type="Signed  (2's comp)"  n_bits=18  bin_pt=17  float_type=Single  exp_bits=8  fraction_bits=24  quantization="Round  (unbiased: +/- Inf)"  overflow=Saturate  en=off  latency=1  dbl_ovrd=off  pipeline=on  block_type=convert
  mults : Subsystem
  c : Outport
  wires:
  a_input_c_to_ri/1(re) -> mults/7(a4), mults/1(a1)  "a_re"
  b_input_c_to_ri/1(re) -> mults/6(b3), mults/2(b1)  "b_re"
  a_input_c_to_ri/2(im) -> mults/5(a3), mults/3(a2)  "a_im"
  b_input_c_to_ri/2(im) -> mults/8(b4), mults/4(b2)  "b_im"
  convert1/1 -> c_output_ri_to_c/2(im)  "c_im"
  AddSub1/1 -> convert1/1
  convert0/1 -> c_output_ri_to_c/1(re)  "c_re"
  AddSub/1 -> convert0/1
  mults/4(c4) -> AddSub1/2
  mults/3(c3) -> AddSub1/1
  mults/2(c2) -> AddSub/2
  mults/1(c1) -> AddSub/1
  c_output_ri_to_c/1(c) -> c/1
  b/1 -> b_input_c_to_ri/1(c)
  a/1 -> a_input_c_to_ri/1(c)

== system fft_wideband_real/fft_wideband_real/phase_mult/cmult_8 ==
  a : Inport
  b : Inport  Port=2
  AddSub : xbsIndex_r4/AddSub  mode=Subtraction  use_carryin=off  use_carryout=off  en=off  latency=2  precision=Full  arith_type=Unsigned  n_bits=16  bin_pt=14  quantization=Truncate  overflow=Wrap  dbl_ovrd=off  use_behavioral_HDL=on  hw_selection=Fabric  pipelined=off  block_type=addsub
  AddSub1 : xbsIndex_r4/AddSub  mode=Addition  use_carryin=off  use_carryout=off  en=off  latency=2  precision=Full  arith_type=Unsigned  n_bits=16  bin_pt=14  quantization=Truncate  overflow=Wrap  dbl_ovrd=off  use_behavioral_HDL=on  hw_selection=Fabric  pipelined=off  block_type=addsub
  a_input_c_to_ri : Subsystem
      settings: AttributesFormatString=18_17 r/i
  b_input_c_to_ri : Subsystem
      settings: AttributesFormatString=18_17 r/i
  c_output_ri_to_c : Subsystem
  convert0 : xbsIndex_r4/Convert  gui_display_data_type=Fixed-point  arith_type="Signed  (2's comp)"  n_bits=18  bin_pt=17  float_type=Single  exp_bits=8  fraction_bits=24  quantization="Round  (unbiased: +/- Inf)"  overflow=Saturate  en=off  latency=1  dbl_ovrd=off  pipeline=on  block_type=convert
  convert1 : xbsIndex_r4/Convert  gui_display_data_type=Fixed-point  arith_type="Signed  (2's comp)"  n_bits=18  bin_pt=17  float_type=Single  exp_bits=8  fraction_bits=24  quantization="Round  (unbiased: +/- Inf)"  overflow=Saturate  en=off  latency=1  dbl_ovrd=off  pipeline=on  block_type=convert
  mults : Subsystem
  c : Outport
  wires:
  a_input_c_to_ri/1(re) -> mults/7(a4), mults/1(a1)  "a_re"
  b_input_c_to_ri/1(re) -> mults/6(b3), mults/2(b1)  "b_re"
  a_input_c_to_ri/2(im) -> mults/5(a3), mults/3(a2)  "a_im"
  b_input_c_to_ri/2(im) -> mults/8(b4), mults/4(b2)  "b_im"
  convert1/1 -> c_output_ri_to_c/2(im)  "c_im"
  AddSub1/1 -> convert1/1
  convert0/1 -> c_output_ri_to_c/1(re)  "c_re"
  AddSub/1 -> convert0/1
  mults/4(c4) -> AddSub1/2
  mults/3(c3) -> AddSub1/1
  mults/2(c2) -> AddSub/2
  mults/1(c1) -> AddSub/1
  c_output_ri_to_c/1(c) -> c/1
  b/1 -> b_input_c_to_ri/1(c)
  a/1 -> a_input_c_to_ri/1(c)

== system fft_wideband_real/fft_wideband_real/phase_mult/cmult_9 ==
  a : Inport
  b : Inport  Port=2
  AddSub : xbsIndex_r4/AddSub  mode=Subtraction  use_carryin=off  use_carryout=off  en=off  latency=2  precision=Full  arith_type=Unsigned  n_bits=16  bin_pt=14  quantization=Truncate  overflow=Wrap  dbl_ovrd=off  use_behavioral_HDL=on  hw_selection=Fabric  pipelined=off  block_type=addsub
  AddSub1 : xbsIndex_r4/AddSub  mode=Addition  use_carryin=off  use_carryout=off  en=off  latency=2  precision=Full  arith_type=Unsigned  n_bits=16  bin_pt=14  quantization=Truncate  overflow=Wrap  dbl_ovrd=off  use_behavioral_HDL=on  hw_selection=Fabric  pipelined=off  block_type=addsub
  a_input_c_to_ri : Subsystem
      settings: AttributesFormatString=18_17 r/i
  b_input_c_to_ri : Subsystem
      settings: AttributesFormatString=18_17 r/i
  c_output_ri_to_c : Subsystem
  convert0 : xbsIndex_r4/Convert  gui_display_data_type=Fixed-point  arith_type="Signed  (2's comp)"  n_bits=18  bin_pt=17  float_type=Single  exp_bits=8  fraction_bits=24  quantization="Round  (unbiased: +/- Inf)"  overflow=Saturate  en=off  latency=1  dbl_ovrd=off  pipeline=on  block_type=convert
  convert1 : xbsIndex_r4/Convert  gui_display_data_type=Fixed-point  arith_type="Signed  (2's comp)"  n_bits=18  bin_pt=17  float_type=Single  exp_bits=8  fraction_bits=24  quantization="Round  (unbiased: +/- Inf)"  overflow=Saturate  en=off  latency=1  dbl_ovrd=off  pipeline=on  block_type=convert
  mults : Subsystem
  c : Outport
  wires:
  a_input_c_to_ri/1(re) -> mults/7(a4), mults/1(a1)  "a_re"
  b_input_c_to_ri/1(re) -> mults/6(b3), mults/2(b1)  "b_re"
  a_input_c_to_ri/2(im) -> mults/5(a3), mults/3(a2)  "a_im"
  b_input_c_to_ri/2(im) -> mults/8(b4), mults/4(b2)  "b_im"
  convert1/1 -> c_output_ri_to_c/2(im)  "c_im"
  AddSub1/1 -> convert1/1
  convert0/1 -> c_output_ri_to_c/1(re)  "c_re"
  AddSub/1 -> convert0/1
  mults/4(c4) -> AddSub1/2
  mults/3(c3) -> AddSub1/1
  mults/2(c2) -> AddSub/2
  mults/1(c1) -> AddSub/1
  c_output_ri_to_c/1(c) -> c/1
  b/1 -> b_input_c_to_ri/1(c)
  a/1 -> a_input_c_to_ri/1(c)

== system fft_wideband_real/fft_wideband_real/phase_mult/phase10_coeffs ==
  rst : Inport
  Counter : xbsIndex_r4/Counter  cnt_type=Free Running  cnt_to=Inf  operation=Up  start_count=0  cnt_by_val=1  arith_type=Unsigned  n_bits=6  bin_pt=0  load_pin=off  rst=on  en=off  explicit_period=on  period=1  dbl_ovrd=off  use_behavioral_HDL=off  implementation=Fabric  block_type=counter
  Slice : xbsIndex_r4/Slice  nbits=6  boolean_output=off  mode=Upper Bit Location + Width  bit1=0  base1=MSB of Input  bit0=0  base0=LSB of Input  dbl_ovrd=off  block_type=slice
  bram_din_const : xbsIndex_r4/Constant  const=0  gui_display_data_type=Fixed-point  arith_type=Signed (2's comp)  n_bits=18  bin_pt=17  preci_type=Single  exp_width=8  frac_width=24  explicit_period=off  period=1  equ=P=C  opselect=C  inp2=PCIN>>17  opr=+  inp1=P  carry=CIN  dbl_ovrd=off  block_type=constant
  bram_we_const : xbsIndex_r4/Constant  const=0  gui_display_data_type=Fixed-point  arith_type=Boolean  n_bits=16  bin_pt=14  preci_type=Single  exp_width=8  frac_width=24  explicit_period=off  period=1  equ=P=C  opselect=C  inp2=PCIN>>17  opr=+  inp1=P  carry=CIN  dbl_ovrd=off  block_type=constant
  cnt_sign_exta : xbsIndex_r4/Convert  gui_display_data_type=Fixed-point  arith_type=Unsigned  n_bits=10  bin_pt=0  float_type=Single  exp_bits=8  fraction_bits=24  quantization=Truncate  overflow=Wrap  en=off  latency=0  dbl_ovrd=off  pipeline=off  block_type=convert
  cnt_sign_extb : xbsIndex_r4/Convert  gui_display_data_type=Fixed-point  arith_type=Unsigned  n_bits=9  bin_pt=0  float_type=Single  exp_bits=8  fraction_bits=24  quantization=Truncate  overflow=Wrap  en=off  latency=0  dbl_ovrd=off  pipeline=off  block_type=convert
  coeff_mem : xbsIndex_r4/Dual Port RAM  depth=1024  initVector=[1 0.99847412109375 0.993904113769531 0.986305236816406 0.975700378417969 0.962120056152344 0.945610046386719 0.92620849609375 0.90399169921875 0.879013061523438 0.851356506347656 0.82110595703125 0.788345336914062 0.753189086914062 0.715728759765625 0.676094055175781 0.634391784667969 0.59075927734375 0.545326232910156 0.49822998046875 0.449607849121094 0.399627685546875 0.348419189453125 0.296150207519531 0.24298095703125 0.189071655273438 0.13458251953125 0.079681396484375 0.0245437622070312 -0.0306777954101562 -0.0858001708984375 -0.140655517578125 -0.195091247558594 -0.248924255371094 -0.302009582519531 -0.354164123535156 -0.405242919921875 -0.455085754394531 -0.5035400390625 -0.550460815429688 -0.595695495605469 -0.639122009277344 -0.68060302734375 -0.720001220703125 -0.757209777832031 -0.792106628417969 -0.824592590332031 -0.854560852050781 -0.881919860839844 -0.906593322753906 -0.928504943847656 -0.947586059570312 -0.963775634765625 -0.977027893066406 -0.9873046875 -0.99456787109375 -0.998794555664062 -0.999984741210938 -0.998115539550781 -0.993209838867188 -0.985275268554688 -0.974342346191406 -0.960433959960938 -0.943595886230469 0 0 0 0 0 0 0 0 0 0 0 0 0 0 0 0 0 0 0 0 0 0 0 0 0 0 0 0 0 0 0 0 0 0 0 0 0 0 0 0 0 0 0 0 0 0 0 0 0 0 0 0 0 0 0 0 0 0 0 0 0 0 0 0 0 0 0 0 0 0 0 0 0 0 0 0 0 0 0 0 0 0 0 0 0 0 0 0 0 0 0 0 0 0 0 0 0 0 0 0 0 0 0 0 0 0 0 0 0 0 0 0 0 0 0 0 0 0 0 0 0 0 0 0 0 0 0 0 0 0 0 0 0 0 0 0 0 0 0 0 0 0 0 0 0 0 0 0 0 0 0 0 0 0 0 0 0 0 0 0 0 0 0 0 0 0 0 0 0 0 0 0 0 0 0 0 0 0 0 0 0 0 0 0 0 0 0 0 0 0 0 0 0 0 0 0 0 0 0 0 0 0 0 0 0 0 0 0 0 0 0 0 0 0 0 0 0 0 0 0 0 0 0 0 0 0 0 0 0 0 0 0 0 0 0 0 0 0 0 0 0 0 0 0 0 0 0 0 0 0 0 0 0 0 0 0 0 0 0 0 0 0 0 0 0 0 0 0 0 0 0 0 0 0 0 0 0 0 0 0 0 0 0 0 0 0 0 0 0 0 0 0 0 0 0 0 0 0 0 0 0 0 0 0 0 0 0 0 0 0 0 0 0 0 0 0 0 0 0 0 0 0 0 0 0 0 0 0 0 0 0 0 0 0 0 0 0 0 0 0 0 0 0 0 0 0 0 0 0 0 0 0 0 0 0 0 0 0 0 0 0 0 0 0 0 0 0 0 0 0 0 0 0 0 0 0 0 0 0 0 0 0 0 0 0 0 0 0 0 0 0 0 0 0 0 0 0 0 0 0 0 0 0 0 0 0 0 0 0 0 0 0 0 0 0 0 0 0 0 0 0 0 0 0 0 0 0 0 0 0 0 0 0 0 0 0 0 0 0 0 0 0 0 0 0 0 0 0 0 -0.0551986694335938 -0.110221862792969 -0.164909362792969 -0.219100952148438 -0.272621154785156 -0.325309753417969 -0.377006530761719 -0.427558898925781 -0.476799011230469 -0.524589538574219 -0.570777893066406 -0.615234375 -0.657806396484375 -0.698379516601562 -0.73681640625 -0.77301025390625 -0.806846618652344 -0.838226318359375 -0.867042541503906 -0.893226623535156 -0.916679382324219 -0.937339782714844 -0.95513916015625 -0.97003173828125 -0.981964111328125 -0.99090576171875 -0.996818542480469 -0.999702453613281 -0.999526977539062 -0.996315002441406 -0.990058898925781 -0.980781555175781 -0.968521118164062 -0.95330810546875 -0.9351806640625 -0.914207458496094 -0.890449523925781 -0.863975524902344 -0.834861755371094 -0.803207397460938 -0.76910400390625 -0.732650756835938 -0.6939697265625 -0.653175354003906 -0.610382080078125 -0.56573486328125 -0.519355773925781 -0.471397399902344 -0.4219970703125 -0.371315002441406 -0.319503784179688 -0.266716003417969 -0.213111877441406 -0.158859252929688 -0.104118347167969 -0.0490646362304688 0.006134033203125 0.0613174438476562 0.116317749023438 0.17095947265625 0.225082397460938 0.278518676757812 0.331108093261719 0 0 0 0 0 0 0 0 0 0 0 0 0 0 0 0 0 0 0 0 0 0 0 0 0 0 0 0 0 0 0 0 0 0 0 0 0 0 0 0 0 0 0 0 0 0 0 0 0 0 0 0 0 0 0 0 0 0 0 0 0 0 0 0 0 0 0 0 0 0 0 0 0 0 0 0 0 0 0 0 0 0 0 0 0 0 0 0 0 0 0 0 0 0 0 0 0 0 0 0 0 0 0 0 0 0 0 0 0 0 0 0 0 0 0 0 0 0 0 0 0 0 0 0 0 0 0 0 0 0 0 0 0 0 0 0 0 0 0 0 0 0 0 0 0 0 0 0 0 0 0 0 0 0 0 0 0 0 0 0 0 0 0 0 0 0 0 0 0 0 0 0 0 0 0 0 0 0 0 0 0 0 0 0 0 0 0 0 0 0 0 0 0 0 0 0 0 0 0 0 0 0 0 0 0 0 0 0 0 0 0 0 0 0 0 0 0 0 0 0 0 0 0 0 0 0 0 0 0 0 0 0 0 0 0 0 0 0 0 0 0 0 0 0 0 0 0 0 0 0 0 0 0 0 0 0 0 0 0 0 0 0 0 0 0 0 0 0 0 0 0 0 0 0 0 0 0 0 0 0 0 0 0 0 0 0 0 0 0 0 0 0 0 0 0 0 0 0 0 0 0 0 0 0 0 0 0 0 0 0 0 0 0 0 0 0 0 0 0 0 0 0 0 0 0 0 0 0 0 0 0 0 0 0 0 0 0 0 0 0 0 0 0 0 0 0 0 0 0 0 0 0 0 0 0 0 0 0 0 0 0 0 0 0 0 0 0 0 0 0 0 0 0 0 0 0 0 0 0 0 0 0 0 0 0 0 0 0 0 0 0 0 0 0 0 0 0 0 0 0 0 0 0 0 0 0 0 0 0 0 0 0 0 0 0 0 0 0 0 0 0 0 0 0 0 0 0 0 0 0 0 0 0 0 0 0 0 0 0 0 0 0 0 0 0 0 0 0]  distributed_mem=Block RAM  init_a=0  init_b=0  rst_a=off  rst_b=off  en_a=off  en_b=off  latency=2  write_mode_A=Read After Write  write_mode_B=Read After Write  dbl_ovrd=off  optimize=Area  use_rpm=on  block_type=dpram
  counter_b_concat : xbsIndex_r4/Concat  num_inputs=2  dbl_ovrd=off  block_type=concat
  counter_b_pad : xbsIndex_r4/Constant  const=1  gui_display_data_type=Fixed-point  arith_type=Unsigned  n_bits=1  bin_pt=0  preci_type=Single  exp_width=8  frac_width=24  explicit_period=off  period=1  equ=P=C  opselect=C  inp2=PCIN>>17  opr=+  inp1=P  carry=CIN  dbl_ovrd=off  block_type=constant
  ri_to_c : Subsystem
  w : Outport
  wires:
  Slice/1 -> cnt_sign_extb/1, cnt_sign_exta/1
  bram_din_const/1 -> coeff_mem/5, coeff_mem/2
  bram_we_const/1 -> coeff_mem/6, coeff_mem/3
  ri_to_c/1(c) -> w/1
  coeff_mem/2 -> ri_to_c/2(im)
  coeff_mem/1 -> ri_to_c/1(re)
  counter_b_concat/1 -> coeff_mem/4
  cnt_sign_exta/1 -> coeff_mem/1
  cnt_sign_extb/1 -> counter_b_concat/2
  counter_b_pad/1 -> counter_b_concat/1
  Counter/1 -> Slice/1
  rst/1 -> Counter/1

== system fft_wideband_real/fft_wideband_real/phase_mult/phase11_coeffs ==
  rst : Inport
  Counter : xbsIndex_r4/Counter  cnt_type=Free Running  cnt_to=Inf  operation=Up  start_count=0  cnt_by_val=1  arith_type=Unsigned  n_bits=6  bin_pt=0  load_pin=off  rst=on  en=off  explicit_period=on  period=1  dbl_ovrd=off  use_behavioral_HDL=off  implementation=Fabric  block_type=counter
  Slice : xbsIndex_r4/Slice  nbits=6  boolean_output=off  mode=Upper Bit Location + Width  bit1=0  base1=MSB of Input  bit0=0  base0=LSB of Input  dbl_ovrd=off  block_type=slice
  bram_din_const : xbsIndex_r4/Constant  const=0  gui_display_data_type=Fixed-point  arith_type=Signed (2's comp)  n_bits=18  bin_pt=17  preci_type=Single  exp_width=8  frac_width=24  explicit_period=off  period=1  equ=P=C  opselect=C  inp2=PCIN>>17  opr=+  inp1=P  carry=CIN  dbl_ovrd=off  block_type=constant
  bram_we_const : xbsIndex_r4/Constant  const=0  gui_display_data_type=Fixed-point  arith_type=Boolean  n_bits=16  bin_pt=14  preci_type=Single  exp_width=8  frac_width=24  explicit_period=off  period=1  equ=P=C  opselect=C  inp2=PCIN>>17  opr=+  inp1=P  carry=CIN  dbl_ovrd=off  block_type=constant
  cnt_sign_exta : xbsIndex_r4/Convert  gui_display_data_type=Fixed-point  arith_type=Unsigned  n_bits=10  bin_pt=0  float_type=Single  exp_bits=8  fraction_bits=24  quantization=Truncate  overflow=Wrap  en=off  latency=0  dbl_ovrd=off  pipeline=off  block_type=convert
  cnt_sign_extb : xbsIndex_r4/Convert  gui_display_data_type=Fixed-point  arith_type=Unsigned  n_bits=9  bin_pt=0  float_type=Single  exp_bits=8  fraction_bits=24  quantization=Truncate  overflow=Wrap  en=off  latency=0  dbl_ovrd=off  pipeline=off  block_type=convert
  coeff_mem : xbsIndex_r4/Dual Port RAM  depth=1024  initVector=[1 0.998115539550781 0.992477416992188 0.983108520507812 0.97003173828125 0.95330810546875 0.932991027832031 0.909164428710938 0.881919860839844 0.851356506347656 0.817581176757812 0.780738830566406 0.740951538085938 0.698379516601562 0.653175354003906 0.605514526367188 0.555572509765625 0.5035400390625 0.449607849121094 0.393989562988281 0.336891174316406 0.278518676757812 0.219100952148438 0.158859252929688 0.0980148315429688 0.03680419921875 -0.0245437622070312 -0.0858001708984375 -0.146728515625 -0.207115173339844 -0.266716003417969 -0.325309753417969 -0.382682800292969 -0.438613891601562 -0.492897033691406 -0.545326232910156 -0.595695495605469 -0.643829345703125 -0.689537048339844 -0.732650756835938 -0.77301025390625 -0.810455322265625 -0.844856262207031 -0.876068115234375 -0.90399169921875 -0.928504943847656 -0.949531555175781 -0.96697998046875 -0.980781555175781 -0.99090576171875 -0.997291564941406 -0.999923706054688 -0.998794555664062 -0.993904113769531 -0.985275268554688 -0.972938537597656 -0.956939697265625 -0.937339782714844 -0.914207458496094 -0.887641906738281 -0.85772705078125 -0.824592590332031 -0.788345336914062 -0.749137878417969 0 0 0 0 0 0 0 0 0 0 0 0 0 0 0 0 0 0 0 0 0 0 0 0 0 0 0 0 0 0 0 0 0 0 0 0 0 0 0 0 0 0 0 0 0 0 0 0 0 0 0 0 0 0 0 0 0 0 0 0 0 0 0 0 0 0 0 0 0 0 0 0 0 0 0 0 0 0 0 0 0 0 0 0 0 0 0 0 0 0 0 0 0 0 0 0 0 0 0 0 0 0 0 0 0 0 0 0 0 0 0 0 0 0 0 0 0 0 0 0 0 0 0 0 0 0 0 0 0 0 0 0 0 0 0 0 0 0 0 0 0 0 0 0 0 0 0 0 0 0 0 0 0 0 0 0 0 0 0 0 0 0 0 0 0 0 0 0 0 0 0 0 0 0 0 0 0 0 0 0 0 0 0 0 0 0 0 0 0 0 0 0 0 0 0 0 0 0 0 0 0 0 0 0 0 0 0 0 0 0 0 0 0 0 0 0 0 0 0 0 0 0 0 0 0 0 0 0 0 0 0 0 0 0 0 0 0 0 0 0 0 0 0 0 0 0 0 0 0 0 0 0 0 0 0 0 0 0 0 0 0 0 0 0 0 0 0 0 0 0 0 0 0 0 0 0 0 0 0 0 0 0 0 0 0 0 0 0 0 0 0 0 0 0 0 0 0 0 0 0 0 0 0 0 0 0 0 0 0 0 0 0 0 0 0 0 0 0 0 0 0 0 0 0 0 0 0 0 0 0 0 0 0 0 0 0 0 0 0 0 0 0 0 0 0 0 0 0 0 0 0 0 0 0 0 0 0 0 0 0 0 0 0 0 0 0 0 0 0 0 0 0 0 0 0 0 0 0 0 0 0 0 0 0 0 0 0 0 0 0 0 0 0 0 0 0 0 0 0 0 0 0 0 0 0 0 0 0 0 0 0 0 0 0 0 0 0 0 0 0 0 0 0 0 0 0 0 0 0 0 0 0 0 0 0 0 0 0 0 0 0 0 0 0 0 0 0 0 0 -0.0613174438476562 -0.122413635253906 -0.183036804199219 -0.24298095703125 -0.302009582519531 -0.359893798828125 -0.416427612304688 -0.471397399902344 -0.524589538574219 -0.5758056640625 -0.624862670898438 -0.671562194824219 -0.715728759765625 -0.757209777832031 -0.79583740234375 -0.831466674804688 -0.863975524902344 -0.893226623535156 -0.919113159179688 -0.941543579101562 -0.960433959960938 -0.975700378417969 -0.9873046875 -0.995185852050781 -0.999320983886719 -0.999702453613281 -0.996315002441406 -0.989173889160156 -0.978317260742188 -0.963775634765625 -0.945610046386719 -0.923881530761719 -0.898674011230469 -0.870086669921875 -0.838226318359375 -0.803207397460938 -0.765167236328125 -0.724250793457031 -0.68060302734375 -0.634391784667969 -0.585800170898438 -0.534996032714844 -0.482185363769531 -0.427558898925781 -0.371315002441406 -0.313682556152344 -0.254867553710938 -0.195091247558594 -0.13458251953125 -0.0735626220703125 -0.01226806640625 0.0490646362304688 0.110221862792969 0.17095947265625 0.231056213378906 0.290283203125 0.348419189453125 0.405242919921875 0.460540771484375 0.51409912109375 0.56573486328125 0.615234375 0.66241455078125 0 0 0 0 0 0 0 0 0 0 0 0 0 0 0 0 0 0 0 0 0 0 0 0 0 0 0 0 0 0 0 0 0 0 0 0 0 0 0 0 0 0 0 0 0 0 0 0 0 0 0 0 0 0 0 0 0 0 0 0 0 0 0 0 0 0 0 0 0 0 0 0 0 0 0 0 0 0 0 0 0 0 0 0 0 0 0 0 0 0 0 0 0 0 0 0 0 0 0 0 0 0 0 0 0 0 0 0 0 0 0 0 0 0 0 0 0 0 0 0 0 0 0 0 0 0 0 0 0 0 0 0 0 0 0 0 0 0 0 0 0 0 0 0 0 0 0 0 0 0 0 0 0 0 0 0 0 0 0 0 0 0 0 0 0 0 0 0 0 0 0 0 0 0 0 0 0 0 0 0 0 0 0 0 0 0 0 0 0 0 0 0 0 0 0 0 0 0 0 0 0 0 0 0 0 0 0 0 0 0 0 0 0 0 0 0 0 0 0 0 0 0 0 0 0 0 0 0 0 0 0 0 0 0 0 0 0 0 0 0 0 0 0 0 0 0 0 0 0 0 0 0 0 0 0 0 0 0 0 0 0 0 0 0 0 0 0 0 0 0 0 0 0 0 0 0 0 0 0 0 0 0 0 0 0 0 0 0 0 0 0 0 0 0 0 0 0 0 0 0 0 0 0 0 0 0 0 0 0 0 0 0 0 0 0 0 0 0 0 0 0 0 0 0 0 0 0 0 0 0 0 0 0 0 0 0 0 0 0 0 0 0 0 0 0 0 0 0 0 0 0 0 0 0 0 0 0 0 0 0 0 0 0 0 0 0 0 0 0 0 0 0 0 0 0 0 0 0 0 0 0 0 0 0 0 0 0 0 0 0 0 0 0 0 0 0 0 0 0 0 0 0 0 0 0 0 0 0 0 0 0 0 0 0 0 0 0 0 0 0 0 0 0 0 0 0 0 0 0 0 0 0 0 0 0 0 0 0 0 0 0 0 0 0 0 0 0 0]  distributed_mem=Block RAM  init_a=0  init_b=0  rst_a=off  rst_b=off  en_a=off  en_b=off  latency=2  write_mode_A=Read After Write  write_mode_B=Read After Write  dbl_ovrd=off  optimize=Area  use_rpm=on  block_type=dpram
  counter_b_concat : xbsIndex_r4/Concat  num_inputs=2  dbl_ovrd=off  block_type=concat
  counter_b_pad : xbsIndex_r4/Constant  const=1  gui_display_data_type=Fixed-point  arith_type=Unsigned  n_bits=1  bin_pt=0  preci_type=Single  exp_width=8  frac_width=24  explicit_period=off  period=1  equ=P=C  opselect=C  inp2=PCIN>>17  opr=+  inp1=P  carry=CIN  dbl_ovrd=off  block_type=constant
  ri_to_c : Subsystem
  w : Outport
  wires:
  Slice/1 -> cnt_sign_extb/1, cnt_sign_exta/1
  bram_din_const/1 -> coeff_mem/5, coeff_mem/2
  bram_we_const/1 -> coeff_mem/6, coeff_mem/3
  ri_to_c/1(c) -> w/1
  coeff_mem/2 -> ri_to_c/2(im)
  coeff_mem/1 -> ri_to_c/1(re)
  counter_b_concat/1 -> coeff_mem/4
  cnt_sign_exta/1 -> coeff_mem/1
  cnt_sign_extb/1 -> counter_b_concat/2
  counter_b_pad/1 -> counter_b_concat/1
  Counter/1 -> Slice/1
  rst/1 -> Counter/1
